simulink model "Hysterisis_current_control"  (R2025a)
settings: Solver=VariableStepAuto  StartTime=0.0  StopTime=5  RelTol=1e-3
libraries: spsIGBTDiodeLib x6, spsDCVoltageSourceLib x1, autolibshared x1, spsGroundLib x1, spsVoltageMeasurementLib x1, spsPermanentMagnetSynchronousMachineLib x1, spsThreePhaseVIMeasurementLib x1, spsUniversalBridgeLib x1, sps_lib x1
settings Model: Creator=mugun  LastModifiedBy=mugun

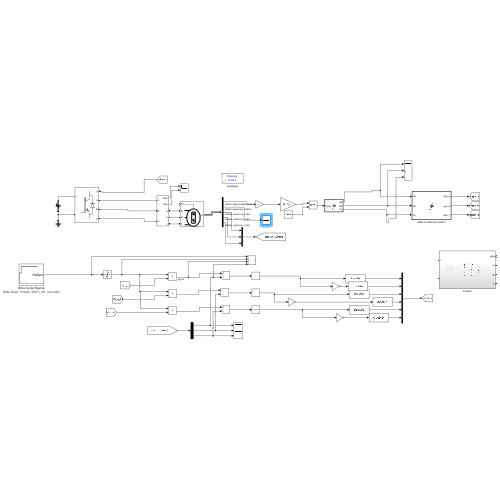
[thumbnail: Simulink's stored preview of the top-level diagram]
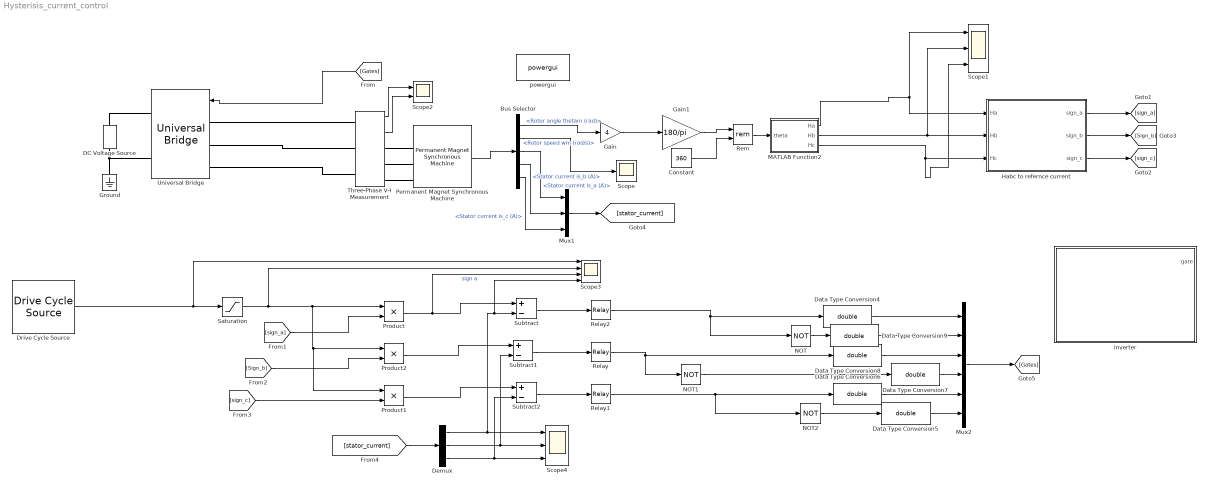
== system Hysterisis_current_control ==
  Bus Selector : BusSelector  OutputSignals=Rotor angle thetam (rad),Rotor speed wm (rad/s),Stator current is_a (A),Stator current is_b (A),Stator current is_c (A)
  Constant : Constant  Value=360
  DC Voltage Source : spsDCVoltageSourceLib/DC Voltage Source  Amplitude=400  Measurements=None
  Data Type Conversion{4..9} (6 alike) : DataTypeConversion  OutDataTypeStr=double  SaturateOnIntegerOverflow=off  RndMeth=Floor
  Demux : Demux  Outputs=3
  Drive Cycle Source : autolibshared/Drive Cycle Source  cycleVar=Wide Open Throttle (WOT)  fileVar=cycleFTP75.mat  tfinal="30  seconds"  cycleRepeat=off  outAccPort=off  outGearPort=off  gearList=No gear data  t_wot1=0.2  xdot_woto=0  xdot_wot1=30  t_wot2=3  xdot_wot2=50  t_wotend=30  srcUnit=m/s  outUnit=m/s  srcAccUnit=m/s/s  outAccUnit=m/s^2  dt=0  aMode=2  faultOption=off  velBnd=2  velBndUnit=mph  inUnit=m/s  timeBnd=1  failOption=off  stopSim=off  maxFaultCnt=10  maxFaultTime=2  maxTotFaultTime=15  traceOption=off  dtTrace=1  traceWindow=10  lastDCname=FTP75  lastOutUnit=mph  lastDT=0  lastTB=1  lastSB=2  forceCalcBound=off
      settings: LibrarySourceBlock=vehdynlibscenario/Drive Cycle Source
  Gain : Gain  Gain=4
  Gain1 : Gain  Gain=180/pi
  Ground : spsGroundLib/Ground  LConnTagsString=a
  Habc to refernce current : MATLAB Function  TreatAsAtomicUnit=on
  Inverter : Subsystem
      settings: PortSchema="{\"entries\":[{\"content\":{\"sides\":[{\"content\":{\"connectorIds\":[\"LConn1\",\"LConn2\"]},\"type\":\"ConnectorPlacement.EquallySpacedRectSide\",\"uuid\":\"18219423-8b1f-43e6-a43a-6c4945a1488d\"},{\"content\":{\"connectorIds\":[\"In1\",\"RConn1\",\"RConn2\",\"RConn3\"],\"side\":\"RIGHT\"},\"type\":\"ConnectorPlacement.EquallySpacedRectSide\",\"uuid\":\"d63a9969-6ec8-4e38-b2d2-b97f72faf8f7\"},{\"content\":{\"side\":\"TOP\"},\"type\":\"ConnectorPlacement.EquallySpacedRectSide\",\"uuid\":\"5719017d-d8ee-42b1-98fe-ac6ef4c4d1f0\"}]},\"type\":\"ConnectorPlacement.EquallySpacedConnector\",\"uuid\":\"d6ba9602-361d-4528-9af6-3ebb689ccd27\"}],\"packageUris\":[\"http://schema.mathworks.com/mf0/Connector/R2020b\"],\"version\":\"1.0\"}"
  MATLAB Function2 : MATLAB Function  TreatAsAtomicUnit=on
  Mux1 : Mux  Inputs=3
  Mux2 : Mux  Inputs=6
  NOT : Logic  Operator=NOT  IconShape=distinctive  AllPortsSameDT=off  OutDataTypeStr=boolean
  NOT1 : Logic  Operator=NOT  IconShape=distinctive  AllPortsSameDT=off  OutDataTypeStr=boolean
  NOT2 : Logic  Operator=NOT  IconShape=distinctive  AllPortsSameDT=off  OutDataTypeStr=boolean
  Permanent Magnet Synchronous Machine : spsPermanentMagnetSynchronousMachineLib/Permanent Magnet Synchronous Machine  NbPhases=3  FluxDistribution=Trapezoidal  RotorType=Round  MechanicalLoad=Torque Tm  PresetModel=No  ShowDetailedParameters=on  MeasurementBus=off  Resistance=0.0485  Inductance=8.5e-3  dqInductances=[8.5e-3,8.5e-3]  La=0.000395  MachineConstant=Flux linkage established by magnets (V.s)  Flux=0.1194  VoltageCst=100.0283  TorqueCst=0.9552  Flat=120  Mechanical=[0.0027 0.0004924 4 0]  PolePairs=4  InitialConditions=[0,0, 0,0]  InitialConditions5ph=[0 0 0 0 0 0]  RefAngle=90 degrees behind phase A axis (modified Park)  IterativeDiscreteModel=Trapezoidal non iterative  TsBlock=-1  TsPowergui=0
  Product : Product
  Product1 : Product
  Product2 : Product
  Relay : Relay  OnSwitchValue=0.01  OffSwitchValue=-0.01
  Relay1 : Relay  OnSwitchValue=0.01  OffSwitchValue=-0.01
  Relay2 : Relay  OnSwitchValue=0.01  OffSwitchValue=-0.01
  Rem : Math  Operator=rem
  Saturation : Saturate  UpperLimit=1  LowerLimit=0
  Scope : Scope
      settings: ActiveDisplayYMinimum=-54.880713457230058  ActiveDisplayYMaximum=493.92642111507064
  Scope1 : Scope  NumInputPorts=3
      settings: ActiveDisplayYMinimum=-1  ActiveDisplayYMaximum=1  DataLoggingVariableName=ScopeData4
  Scope2 : Scope  NumInputPorts=2
      settings: ActiveDisplayYMinimum=-12.545022908119766  ActiveDisplayYMaximum=112.54270150537322  DataLoggingVariableName=ScopeData2
  Scope3 : Scope  NumInputPorts=4
      settings: ActiveDisplayYMinimum=-37.499999999999993  ActiveDisplayYMaximum=337.5  DataLoggingVariableName=ScopeData5
  Scope4 : Scope  NumInputPorts=3
      settings: ActiveDisplayYMinimum=-5.062472900859726  ActiveDisplayYMaximum=4.9191108543194  DataLoggingVariableName=ScopeData7
  Subtract : Sum  Inputs=+-
  Subtract1 : Sum  Inputs=+-
  Subtract2 : Sum  Inputs=+-
  Three-Phase V-I Measurement : spsThreePhaseVIMeasurementLib/Three-Phase V-I Measurement  VoltageMeasurement=phase-to-ground  SetLabelV=off  LabelV=Vabc  Vpu=off  VpuLL=off  CurrentMeasurement=yes  SetLabelI=off  LabelI=Iabc  Ipu=off  Pbase=100e6  Vbase=500e3  OutputType=Complex  PhasorSimulation=off  PSBequivalent=0
  Universal Bridge : spsUniversalBridgeLib/Universal Bridge  Arms=3  SnubberResistance=1e5  SnubberCapacitance=inf  Device=IGBT / Diodes  Ron=1e-3  Lon=0  ForwardVoltages="[  0  0  ]"  ForwardVoltage=0  GTOparameters=[ 10e-6 , 20e-6 ]  IGBTparameters=[ 1e-6 , 2e-6 ]  Measurements=None  Measurements_2=None  converterType=Rectifier
  powergui : sps_lib/powergui  Priority=1  SimulationMode=Discrete  SampleTime=1e-6  frequency=60  Iterations=50  frequencyindice=0  Pbase=100e6  ErrMax=1e-4  UnitsV=kV  UnitsW=MW  buscounter=0  FunctionMessages=off  echomessages=off  EnableUseOfTLC=off  CurrentSourceSwitches=off  DisableSnubberDevices=off  DisableRonSwitches=off  DisableVfSwitches=off  DisplayEquations=off  AutomaticDiscreteSolvers=off  SolverType=Tustin/Backward Euler (TBE)  Interpol=off  ExternalGateDelay=off  methode=off  Ts=100  x0status=blocks  SPID=on  SwTol=0  HookPort=off  NonlinearTolerance=1e-4  nMaxIteration=100  ContinueOnMaxIteration=off  RestoreLinks=warning  ResistiveCurrentMeasurement=off  Frange=[0:2:500]  Ylog=off  Xlog=on  ShowGrid=off  save=off  variable=ZData  structure=0  ZoomFFT=off  StartTime=0.0  cycles=1  DisplayStyle=1  fundamental=60  FreqAxis=off  MaxFrequency=1000  frequencyindicesteady=1  RmsSteady=1  display=off
  wires:
  Permanent Magnet Synchronous Machine/1 -> Bus Selector/1
  Bus Selector/1 -> Gain/1  "<Rotor angle thetam (rad)>"
  Gain/1 -> Gain1/1
  Gain1/1 -> Rem/1
  Constant/1 -> Rem/2
  Rem/1 -> MATLAB Function2/1(theta)
  Bus Selector/2 -> Scope/1  "<Rotor speed wm (rad/s)>"
  Three-Phase V-I Measurement/1 -> Scope2/1
  Three-Phase V-I Measurement/2 -> Scope2/2
  [Gates] -> Universal Bridge/1
  MATLAB Function2/1(Ha) -> Scope1/1, Habc to refernce current/1(Ha)
  MATLAB Function2/2(Hb) -> Scope1/2, Habc to refernce current/2(Hb)
  MATLAB Function2/3(Hc) -> Scope1/3, Habc to refernce current/3(Hc)
  Habc to refernce current/1(sign_a) -> [sign_a]
  Habc to refernce current/2(sign_b) -> [Sign_b]
  Habc to refernce current/3(sign_c) -> [sign_c]
  Drive Cycle Source/1 -> Scope3/1, Saturation/1
  Saturation/1 -> Scope3/2, Product1/1, Product2/1, Product/1
  [sign_a] -> Product/2
  [Sign_b] -> Product2/2
  [sign_c] -> Product1/2
  Bus Selector/3 -> Mux1/1  "<Stator current is_a (A)>"
  Bus Selector/4 -> Mux1/2  "<Stator current is_b (A)>"
  Bus Selector/5 -> Mux1/3  "<Stator current is_c (A)>"
  Mux1/1 -> [stator_current]
  Product/1 -> Scope3/3, Subtract/1  "sign a"
  Product2/1 -> Subtract1/1
  Product1/1 -> Subtract2/1
  [stator_current] -> Demux/1
  Demux/1 -> Scope4/1, Scope3/4, Subtract/2
  Demux/2 -> Scope4/2, Subtract1/2
  Demux/3 -> Scope4/3, Subtract2/2
  Subtract/1 -> Relay2/1
  Subtract1/1 -> Relay/1
  Subtract2/1 -> Relay1/1
  Relay2/1 -> Data Type Conversion4/1, NOT/1
  Relay/1 -> NOT1/1, Data Type Conversion8/1
  Relay1/1 -> NOT2/1, Data Type Conversion6/1
  NOT/1 -> Data Type Conversion9/1
  NOT1/1 -> Data Type Conversion7/1
  NOT2/1 -> Data Type Conversion5/1
  Mux2/1 -> [Gates]
  Data Type Conversion4/1 -> Mux2/1
  Data Type Conversion9/1 -> Mux2/2
  Data Type Conversion8/1 -> Mux2/3
  Data Type Conversion7/1 -> Mux2/4
  Data Type Conversion6/1 -> Mux2/5
  Data Type Conversion5/1 -> Mux2/6
  connections:
  DC Voltage Source/LConn1 -- Universal Bridge/RConn2 -- Ground/LConn1
  Three-Phase V-I Measurement/RConn1 -- Permanent Magnet Synchronous Machine/LConn1
  Three-Phase V-I Measurement/RConn2 -- Permanent Magnet Synchronous Machine/LConn2
  Three-Phase V-I Measurement/RConn3 -- Permanent Magnet Synchronous Machine/LConn3
  Universal Bridge/LConn1 -- Three-Phase V-I Measurement/LConn1
  Universal Bridge/LConn2 -- Three-Phase V-I Measurement/LConn2
  Universal Bridge/LConn3 -- Three-Phase V-I Measurement/LConn3
  Universal Bridge/RConn1 -- DC Voltage Source/RConn1

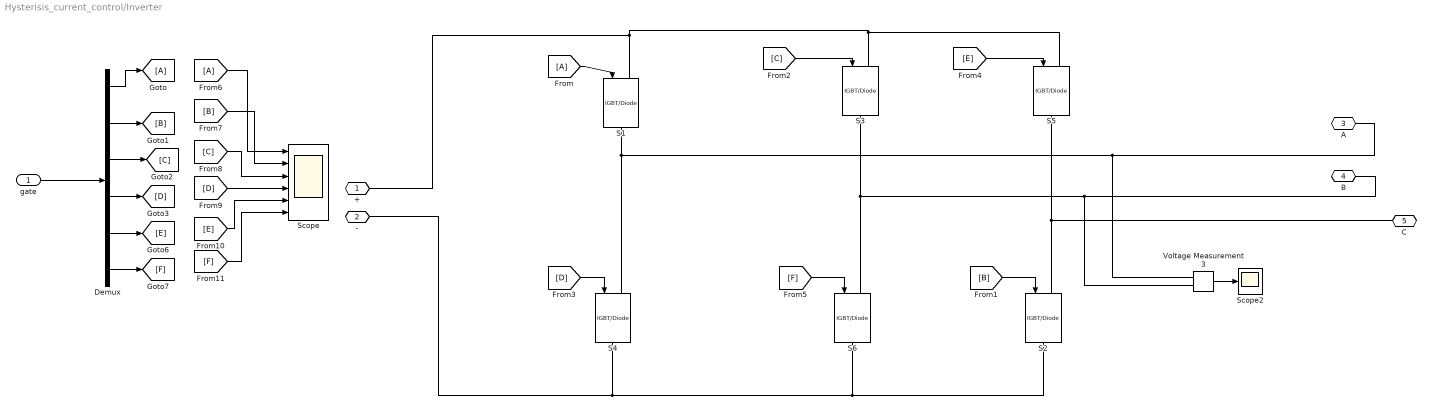
== system Hysterisis_current_control/Inverter ==
  gate : Inport
  Demux : Demux  Outputs=6
  From : From
  From6 : From
  Goto : Goto
  S{1..6} (6 alike) : spsIGBTDiodeLib/IGBT//Diode  Ron=1e-3  Rs=1e5  Cs=inf  Measurements=off
  Scope : Scope  NumInputPorts=6
      settings: ActiveDisplayYMinimum=-0.12499999999999997  ActiveDisplayYMaximum=1.125
  Scope2 : Scope
      settings: ActiveDisplayYMinimum=-125.04211749866226  ActiveDisplayYMaximum=125.01656195858735  DataLoggingVariableName=ScopeData3
  Voltage Measurement3 : spsVoltageMeasurementLib/Voltage Measurement  PhasorSimulation=off  OutputType=Complex  PSBequivalent=0
  + : PMIOPort  Side=Left
  - : PMIOPort  Port=2  Side=Left
  A : PMIOPort  Port=3  Side=Right
  B : PMIOPort  Port=4  Side=Right
  C : PMIOPort  Port=5  Side=Right
  wires:
  [F] -> Scope/6
  From/1 -> S1/1
  [D] -> Scope/4
  [F] -> S6/1
  [C] -> S3/1
  Demux/2 -> [B]
  Demux/1 -> Goto/1
  [D] -> S4/1
  Demux/3 -> [C]
  From6/1 -> Scope/1
  [B] -> Scope/2
  [C] -> Scope/3
  gate/1 -> Demux/1
  [B] -> S2/1
  [E] -> S5/1
  Demux/4 -> [D]
  Demux/5 -> [E]
  [E] -> Scope/5
  Voltage Measurement3/1 -> Scope2/1
  Demux/6 -> [F]
  connections:
  S2/RConn1 -- S6/RConn1 -- -/RConn1 -- S4/RConn1
  Voltage Measurement3/LConn2 -- S3/RConn1 -- S6/LConn1 -- B/RConn1
  S5/RConn1 -- S2/LConn1 -- C/RConn1
  S4/LConn1 -- S1/RConn1 -- A/RConn1 -- Voltage Measurement3/LConn1
  S5/LConn1 -- S3/LConn1 -- S1/LConn1 -- +/RConn1

== matlab function Hysterisis_current_control/Habc to refernce current ==
  data: Ha input; sign_a output; Hb input; Hc input; sign_b output; sign_c output
function [sign_a,sign_b,sign_c] = fcn(Ha,Hb,Hc)

if (Ha==1 && Hb==0 && Hc==1)
    sign_a=1;
    sign_b=0;
    sign_c=-1;

elseif (Ha==1 && Hb==0 && Hc==0)
    sign_a=0;
    sign_b=1;
    sign_c=-1;

elseif (Ha==1 && Hb==1 && Hc==0)
    sign_a=-1;
    sign_b=1;
    sign_c=0;

elseif (Ha==0 && Hb==1 && Hc==0)
    sign_a=-1;
    sign_b=0;
    sign_c=1;

elseif (Ha==0 && Hb==1 && Hc==1)
    sign_a=0;
    sign_b=-1;
    sign_c=1;

elseif (Ha==0 && Hb==0 && Hc==1)
    sign_a=1;
    sign_b=-1;
    sign_c=0;

else 
    sign_a=0;
    sign_b=0;
    sign_c=0;

end

== matlab function Hysterisis_current_control/MATLAB Function2 ==
  data: theta input; Ha output; Hb output; Hc output
function [Ha,Hb,Hc] = fcn(theta)

if (theta>330 && theta<=360) || (theta>=0 && theta<=30)
    Ha=1;
    Hb=0;
    Hc=1;

elseif (theta>30 && theta<=90)
    Ha=1;
    Hb=0;
    Hc=0;
elseif (theta>90 && theta<=150)
    Ha=1;
    Hb=1;
    Hc=0;
elseif (theta>150 && theta<=210)
    Ha=0;
    Hb=1;
    Hc=0;
elseif (theta>210 && theta<=270)
    Ha=0;
    Hb=1;
    Hc=1;
elseif (theta>270 && theta<=330)
    Ha=0;
    Hb=0;
    Hc=1;
else
    Ha=0;
    Hb=0;
    Hc=0;
end
